simulink model "KNN_DataGen"  (R2021b)
settings: Solver=VariableStepAuto  StartTime=0.0  StopTime=1e-8  FixedStep=1e-6  RelTol=1e-3
PreLoadFcn:
  | R = 100;
  | FreqCarrier = 5e9;
  | lambdaCarrier = physconst('lightspeed')/FreqCarrier;
  | 
  | Gt = 7.9988; %[dBi]
  | Gr = Gt; %[dBi]
  | Zin_t =56.2947 - 1j*4.2629; %[Ohm]
  | Zin_r = Zin_t; %[Ohm]
undefined symbols (not defined in the file or in its folder): physconst, S
libraries: simrfV2elements x12, simrfV2util1 x12, rfBudgetAnalyzer_lib x6, simrfV2sources1 x1
settings Model: Creator=The MathWorks, Inc.  LastModifiedBy=Abhinav
settings SolverCC: AlgebraicLoopSolver=TrustRegion
settings DebuggingCC: SFMachineParentedDataDiag=warning

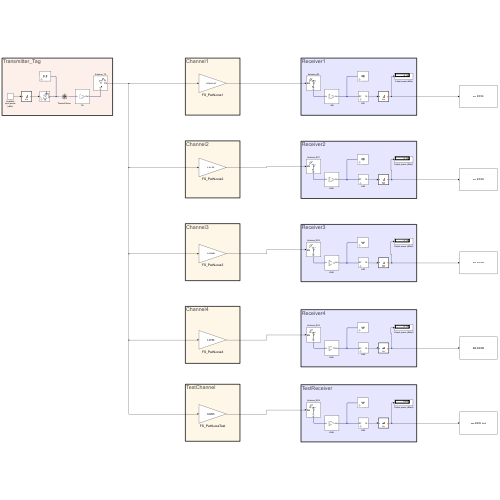
[thumbnail: Simulink's stored preview of the top-level diagram]
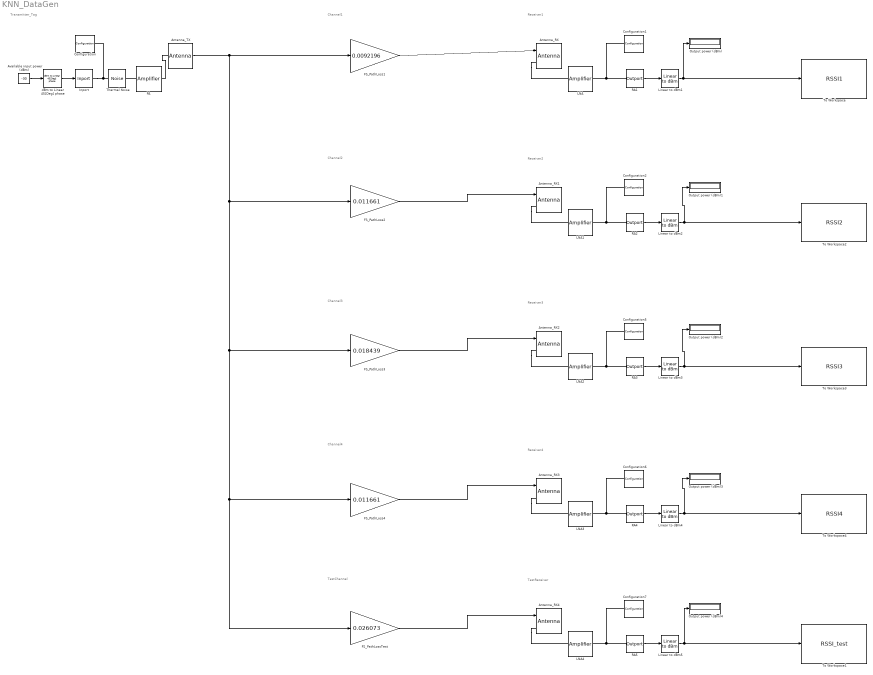
== system KNN_DataGen ==
  note: Channel1
  note: Receiver1
  note: Transmitter_Tag
  note: Channel2
  note: Channel3
  note: Channel4
  note: TestChannel
  note: Receiver2
  note: Receiver3
  note: Receiver4
  note: TestReceiver
  Antenna_RX{,1..4} (5 alike) : simrfV2elements/Antenna  AntennaSource=Isotropic radiator  PrevAppliedAntSource=Isotropic radiator  Gr=6 dBi  Zin=50  AntennaObj=antObj  InputIncWave=on  OutputRadWave=off  CarrierFreqInc=FreqCarrier Hz  rArr=[0 -90] deg  CarrierFreqRad=915000000 GHz  rDep=[0 0] deg  AddNoise=off  InternalGrounding=on  SparamRepresentationImp=Frequency domain  FitTolImp=-80  AutoImpulseLengthImp=off  ImpulseLengthImp=0 s
      settings: SourceProductBaseCode=RB
  Antenna_TX : simrfV2elements/Antenna  AntennaSource=Isotropic radiator  PrevAppliedAntSource=Isotropic radiator  Gr=1.56 dBi  Zin=0.7056465+291.6241i  AntennaObj=antObj  InputIncWave=off  OutputRadWave=on  CarrierFreqInc=2.1 GHz  rArr=[180 0] deg  CarrierFreqRad=915000000 Hz  rDep=[0 90] deg  AddNoise=off  InternalGrounding=on  SparamRepresentationImp=Frequency domain  FitTolImp=-80  AutoImpulseLengthImp=off  ImpulseLengthImp=0 s
      settings: SourceProductBaseCode=RB
  Available input power (dBm) : Constant  Value=-30
  Configuration{,1..2,5..7} (6 alike) : simrfV2util1/Configuration  AutoFreq=on  Tones=[5] GHz  Harmonics=[7]  NormalizeCarrierPower=on  SolverType=Auto  UseCCode=on  StepSize=(1/100000000)/8 s  AddNoise=off  defaultRNG=on  Seed=0  Temperature=290.0 K  SolverDelFlag=0  AbsTol=1e-6  RelTol=1e-3  MaxIter=10  ErrorEstimationType=2-norm over all variables  EnableInterpFilter=on  HiddenFIRfilterControllerParam=on  SmallSignalApprox=off  AllSimFreqs=on  SimFreqs=[] Hz  SimFreqsInternal=[]  SamplesPerFrame=1
      settings: SourceProductBaseCode=RB
  FS_PathLoss1 : Gain  Gain=0.0092196
  FS_PathLoss2 : Gain  Gain=0.011661
  FS_PathLoss3 : Gain  Gain=0.018439
  FS_PathLoss4 : Gain  Gain=0.011661
  FS_PathLossTest : Gain  Gain=0.026073
  Inport : simrfV2util1/Inport  SimulinkInputSignalType=Power  CarrierFreq=915000000 Hz  ZS=50  InternalGrounding=on
      settings: SourceProductBaseCode=RB
  LNA{,1..4} (5 alike) : simrfV2elements/Amplifier  classname=amplifier  DataSource=Data file  File=unitygain.s2p  Paramtype=S-parameters  Sparam=[0 0;1 0]  SparamFreq=1e9 Hz  SparamZ0=50  Residues=0  Poles=0  DF={0 0; 1 0}  Source_linear_gain=Available power gain  linear_gain=20 dB  Zin=50  Zout=50  Source_Poly=Even and odd order  Poly_Coeffs=[0 1]  IPType=Output  IP2=inf dBm  IP3=inf dBm  P1dB=inf dBm  Psat=inf dBm  Gcomp=inf dBm  InternalGrounding=on  SourceFreq=Extracted from data source  PlotFreq=[1e9:1e6:3e9] Hz  PlotType=X-Y plane  YParam1=S(1,1)  YFormat1=Magnitude (decibels)  YParam2=None  YFormat2=Magnitude (decibels)  YOption=Linear  XOption=Linear  SparamRepresentation=Time domain (rationalfit)  FitTol=-40  FitOpt=Fit individually  MaxPoles=48  AutoImpulseLength=on  ImpulseLength=1e-10 s  MagModeling=off  AddNoise=on  NoiseType=Noise figure  NoiseDist=White  NF=0  MinNF=0  Gopt=0  RN=0  CarrierFreq=0 Hz  NoiseAutoImpulseLength=on  NoiseImpulseLength=1e-10 s  SpecifyOpFreq=off  OpFreq=0 Hz
      settings: SourceProductBaseCode=RB
  Linear to dBm{1..5} (5 alike) : rfBudgetAnalyzer_lib/Linear to dBm  SystemSampleTime=-1  VariantActivationTime=update diagram  Latency=0  AutoFrameSizeCalculation=off
      settings: SourceProductBaseCode=RB
  Output power (dBm){,1..4} (5 alike) : Display
  PA : simrfV2elements/Amplifier  classname=amplifier  DataSource=Data file  File=unitygain.s2p  Paramtype=S-parameters  Sparam=[0 0;1 0]  SparamFreq=1e9 Hz  SparamZ0=50  Residues=0  Poles=0  DF={0 0; 1 0}  Source_linear_gain=Available power gain  linear_gain=35 dB  Zin=50  Zout=Zin_t'  Source_Poly=Even and odd order  Poly_Coeffs=[0 1]  IPType=Output  IP2=inf dBm  IP3=inf dBm  P1dB=inf dBm  Psat=inf dBm  Gcomp=inf dBm  InternalGrounding=on  SourceFreq=Extracted from data source  PlotFreq=[1e9:1e6:3e9] Hz  PlotType=X-Y plane  YParam1=S(1,1)  YFormat1=Magnitude (decibels)  YParam2=None  YFormat2=Magnitude (decibels)  YOption=Linear  XOption=Linear  SparamRepresentation=Time domain (rationalfit)  FitTol=-40  FitOpt=Fit individually  MaxPoles=48  AutoImpulseLength=on  ImpulseLength=1e-10 s  MagModeling=off  AddNoise=on  NoiseType=Noise figure  NoiseDist=White  NF=0  MinNF=0  Gopt=0  RN=0  CarrierFreq=0 Hz  NoiseAutoImpulseLength=on  NoiseImpulseLength=1e-10 s  SpecifyOpFreq=off  OpFreq=0 Hz
      settings: SourceProductBaseCode=RB
  RA{1..5} (5 alike) : simrfV2util1/Outport  SensorType=Power  OutputFormat=Complex Baseband  CarrierFreq=915000000 Hz  ZL=50  InternalGrounding=on  StepSize=1e-6 s  AutoStep=on
      settings: SourceProductBaseCode=RB
  Thermal Noise : simrfV2sources1/Noise  SimulinkInputSignalType=Ideal voltage  NoiseType=White  NoisePSD=4*physconst('Boltzmann')*290*50  CarrierFreq=0 Hz  AutoImpulseLength=on  ImpulseLength=1e-10 s  InternalGrounding=off
      settings: SourceProductBaseCode=RB
  To Workspace : ToWorkspace  VariableName=RSSI1  SampleTime=-1
  To Workspace1 : ToWorkspace  VariableName=RSSI_test  SampleTime=-1
  To Workspace2 : ToWorkspace  VariableName=RSSI2  SampleTime=-1
  To Workspace3 : ToWorkspace  VariableName=RSSI3  SampleTime=-1
  To Workspace4 : ToWorkspace  VariableName=RSSI4  SampleTime=-1
  dBm to Linear 45[Deg] phase : rfBudgetAnalyzer_lib/dBm to Linear 45[Deg] phase  SystemSampleTime=-1  VariantActivationTime=update diagram  Latency=0  AutoFrameSizeCalculation=off
      settings: SourceProductBaseCode=RB
  wires:
  Available input power (dBm)/1 -> dBm to Linear 45[Deg] phase/1
  dBm to Linear 45[Deg] phase/1 -> Inport/1
  RA1/1 -> Linear to dBm1/1
  Linear to dBm1/1 -> To Workspace/1, Output power (dBm)/1
  FS_PathLoss1/1 -> Antenna_RX/1
  Antenna_TX/1 -> FS_PathLossTest/1, FS_PathLoss4/1, FS_PathLoss3/1, FS_PathLoss2/1, FS_PathLoss1/1
  RA2/1 -> Linear to dBm2/1
  Linear to dBm2/1 -> To Workspace2/1, Output power (dBm)1/1
  RA3/1 -> Linear to dBm3/1
  Linear to dBm3/1 -> To Workspace3/1, Output power (dBm)2/1
  RA4/1 -> Linear to dBm4/1
  Linear to dBm4/1 -> To Workspace4/1, Output power (dBm)3/1
  RA5/1 -> Linear to dBm5/1
  Linear to dBm5/1 -> To Workspace1/1, Output power (dBm)4/1
  FS_PathLoss2/1 -> Antenna_RX1/1
  FS_PathLoss3/1 -> Antenna_RX2/1
  FS_PathLoss4/1 -> Antenna_RX3/1
  FS_PathLossTest/1 -> Antenna_RX4/1
  connections:
  Configuration/LConn1 -- Inport/RConn1 -- Thermal Noise/RConn1
  PA/LConn1 -- Thermal Noise/LConn1
  RA1/LConn1 -- Configuration1/LConn1 -- LNA/RConn1
  Antenna_RX/LConn1 -- LNA/LConn1
  Antenna_TX/LConn1 -- PA/RConn1
  LNA1/RConn1 -- RA2/LConn1 -- Configuration2/LConn1
  Antenna_RX1/LConn1 -- LNA1/LConn1
  LNA2/RConn1 -- RA3/LConn1 -- Configuration5/LConn1
  Antenna_RX2/LConn1 -- LNA2/LConn1
  LNA3/RConn1 -- RA4/LConn1 -- Configuration6/LConn1
  Antenna_RX3/LConn1 -- LNA3/LConn1
  LNA4/RConn1 -- RA5/LConn1 -- Configuration7/LConn1
  Antenna_RX4/LConn1 -- LNA4/LConn1
